simulink model "dcmotor"  (R2015a)
settings: Solver=ode45  StartTime=0.0  StopTime=10.0  RelTol=1e-3
settings Model: Creator=Aranya Dan  LastModifiedBy=Aranya Dan

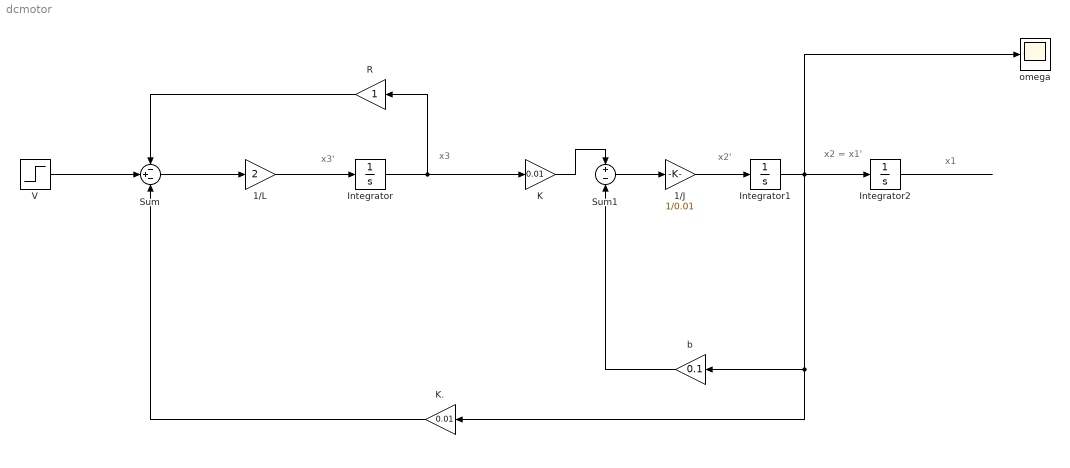
== system dcmotor ==
  note: x1
  note: x2 = x1'
  note: x2'
  note: x3
  note: x3'
  1/J : Gain  Gain=1/0.01
  1/L : Gain  Gain=2
  Integrator : Integrator
  Integrator1 : Integrator
  Integrator2 : Integrator
  K : Gain  Gain=0.01
  K. : Gain  Gain=0.01
  R : Gain
  Sum : Sum  Inputs=-+-
  Sum1 : Sum  Inputs=+-
  V : Step  Time=0  After=10  SampleTime=0
  b : Gain  Gain=0.1
  omega : Scope
  wires:
  Sum/1 -> 1/L/1
  1/L/1 -> Integrator/1
  Integrator/1 -> R/1, K/1
  Sum1/1 -> 1/J/1
  1/J/1 -> Integrator1/1
  Integrator1/1 -> Integrator2/1, omega/1, K./1, b/1
  b/1 -> Sum1/2
  K/1 -> Sum1/1
  V/1 -> Sum/2
  K./1 -> Sum/3
  R/1 -> Sum/1
  Integrator2/1 -> ?
